simulink model "Flightsim2"  (R2024b)
settings: Solver=ode4  StartTime=0  StopTime=100  FixedStep=0.01  RelTol=1e-3
values from neighbouring files (symbols this model uses):
  InitialVel = [f16.state.state(4),f16.state.state(5),f16.state.state(6)]    [MOCK1.m]    (also in simulinkscript.m = initial_state(4:6); trimsolver.m = [f16.state.state(4), f16.state.state(5), f16.state.state(6)])
undefined symbols (not defined in the file or in its folder): aircraft_interface_sim, Earth, f, WGS84
libraries: simulink_extras x3, aerolibfltsims x2, instrumentlib x2, shared6dof x1, aerolibtransform2 x1
settings Model: Creator=naman  LastModifiedBy=naman
settings SolverCC: AlgebraicLoopSolver=LineSearch
settings DataIOCC: SaveState=on

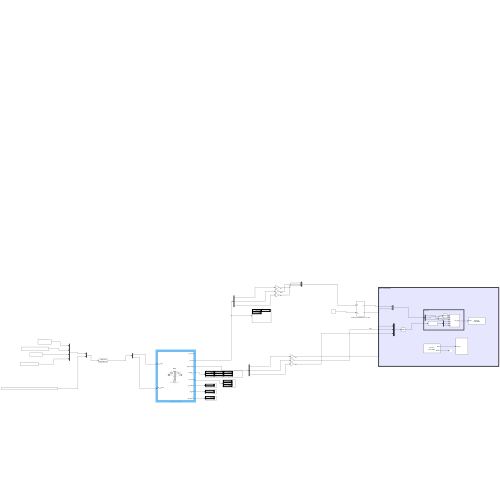
[thumbnail: Simulink's stored preview of the top-level diagram]
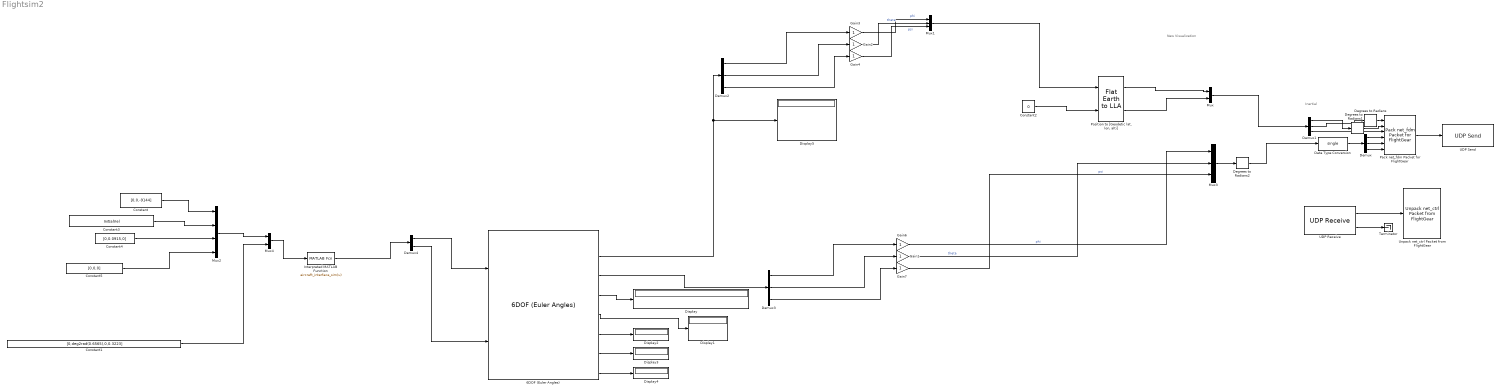
== system Flightsim2 ==
  note: New Visualization
  note: Inertial
  6DOF (Euler Angles) : shared6dof/6DOF (Euler Angles)  units=Metric (MKS)  mtype=Fixed  rep=Euler Angles  xme_0=Initialpos  Vm_0=InitialVel  eul_0=InitialOri  pm_0=InitialRot  mass_0=mass_kg  mass_e=0.5  mass_f=2.0  inertia=Inertia  inertia_e=eye(3)  inertia_f=2*eye(3)  k_quat=1.0  vre_flag=on  abi_flag=off  aMode=0  xme_statename=''  Vm_statename=''  eul_statename=''  quat_statename=''  pm_statename=''  mass_statename=''
  Constant : Constant  Value=[0,0,-9144]
  Constant1 : Constant  Value=[0,deg2rad(0.6565),0,0.3223]
  Constant2 : Constant  Value=0
  Constant3 : Constant  Value=InitialVel
  Constant4 : Constant  Value=[0,0.0915,0]
  Constant5 : Constant  Value=[0,0,0]
  Data Type Conversion : DataTypeConversion  OutDataTypeStr=single  SaturateOnIntegerOverflow=off  RndMeth=Floor
  Degrees to Radians : simulink_extras/Transformations/Degrees to Radians
  Degrees to Radians1 : simulink_extras/Transformations/Degrees to Radians
  Degrees to Radians2 : simulink_extras/Transformations/Degrees to Radians
  Demux{,1..3} (4 alike) : Demux  Outputs=3
  Demux4 : Demux  Outputs=2
  Display{,1..5} (6 alike) : Display
  Gain{1..4,6..7} (6 alike) : Gain
  Interpreted MATLAB Function : MATLABFcn  MATLABFcn=aircraft_interface_sim(u)  OutputDimensions=6
  Mux : Mux  Inputs=2
  Mux1 : Mux  Inputs=3
  Mux2 : Mux
  Mux3 : Mux  Inputs=3
  Mux4 : Mux  Inputs=2
  Pack net_fdm Packet for FlightGear : aerolibfltsims/Pack net_fdm Packet for FlightGear  FlightGearVersion=v2019.1  ShowPositionAttitudeInputs=on  ShowVelocityAccelerationInputs=off  ShowControlSurfacePositionInputs=off  ShowEngineFuelInputs=off  ShowLandingGearInputs=off  ShowEnvironmentInputs=off  SampleTime=-1  packetVersion=24
  "Position to [Geodetic lat, lon, alti]" : aerolibtransform2/Flat Earth to LLA  units=Metric (MKS)  ptype=Earth (WGS84)  F=1/298.257223563  R=6378137  refPosPort=off  LL0=[37.210265015306916, -80.41446644179189]  psi=0
  Terminator : Terminator
  UDP Receive : instrumentlib/UDP Receive  LocalAddress=127.0.0.1  LocalPort=50001  EnablePortSharing=off  Host=localhost  Port=65343  GetLatestData=on  DataSize=[ 1, 744 ]  DataType=uint8  ASCIIFormatting=%f,  Terminator=LF  CustomTerminator=10  ByteOrder=little-endian  EnableBlockingMode=off  Timeout=10  SampleTime=0.2  SimulateUsing=Interpreted execution
  UDP Send : instrumentlib/UDP Send  Host=localhost  Port=50000  LocalAddress=127.0.0.1  LocalPort=-1  EnablePortSharing=on  OutputDatagramPacketSize=4096  ByteOrder=big-endian  EnableBlockingMode=on  SimulateUsing=Interpreted execution
  Unpack net_ctrl Packet from FlightGear : aerolibfltsims/Unpack net_ctrl Packet from FlightGear  FlightGearVersion=v2019.1  ShowControlSurfacePositionOutputs=off  ShowEngineFuelOutputs=off  ShowLandingGearOutputs=off  ShowAvionicOutputs=off  ShowEnvironmentOutputs=off  SampleTime=-1  packetVersion=27
  wires:
  UDP Receive/1 -> Unpack net_ctrl Packet from FlightGear/1
  "Position to [Geodetic lat, lon, alti]"/2 -> Mux/2
  Demux/3 -> Pack net_fdm Packet for FlightGear/6
  Gain1/1 -> Mux3/2  "theta"
  Mux3/1 -> Degrees to Radians2/1
  Demux1/2 -> Degrees to Radians/1
  Degrees to Radians1/1 -> Pack net_fdm Packet for FlightGear/2
  Gain6/1 -> Mux3/1  "phi"
  Data Type Conversion/1 -> Demux/1
  Demux/1 -> Pack net_fdm Packet for FlightGear/4
  Demux/2 -> Pack net_fdm Packet for FlightGear/5
  UDP Receive/2 -> Terminator/1
  "Position to [Geodetic lat, lon, alti]"/1 -> Mux/1
  Demux1/3 -> Pack net_fdm Packet for FlightGear/3
  Gain7/1 -> Mux3/3  "psi"
  Degrees to Radians2/1 -> Data Type Conversion/1
  Pack net_fdm Packet for FlightGear/1 -> UDP Send/1
  Degrees to Radians/1 -> Pack net_fdm Packet for FlightGear/1
  Demux1/1 -> Degrees to Radians1/1
  Mux/1 -> Demux1/1
  6DOF (Euler Angles)/4 -> Display/1
  6DOF (Euler Angles)/3 -> Demux3/1
  Demux3/1 -> Gain6/1
  Demux3/2 -> Gain1/1
  Demux3/3 -> Gain7/1
  6DOF (Euler Angles)/5 -> Display1/1
  6DOF (Euler Angles)/6 -> Display2/1
  6DOF (Euler Angles)/7 -> Display3/1
  6DOF (Euler Angles)/8 -> Display4/1
  Demux2/1 -> Gain3/1
  Demux2/3 -> Gain4/1
  Demux2/2 -> Gain2/1
  6DOF (Euler Angles)/2 -> Demux2/1, Display5/1
  Gain4/1 -> Mux1/3  "psi"
  Gain3/1 -> Mux1/1  "phi"
  Gain2/1 -> Mux1/2  "theta"
  Mux1/1 -> "Position to [Geodetic lat, lon, alti]"/1
  Constant2/1 -> "Position to [Geodetic lat, lon, alti]"/2
  Interpreted MATLAB Function/1 -> Demux4/1
  Mux4/1 -> Interpreted MATLAB Function/1
  Demux4/1 -> 6DOF (Euler Angles)/1
  Demux4/2 -> 6DOF (Euler Angles)/2
  Mux2/1 -> Mux4/1
  Constant/1 -> Mux2/1
  Constant3/1 -> Mux2/2
  Constant4/1 -> Mux2/3
  Constant5/1 -> Mux2/4
  Constant1/1 -> Mux4/2
